simulink model "task4_neo"  (Simulink 8.3)
settings: Solver=ode45  StartTime=0.0  StopTime=250  RelTol=1e-3
PreLoadFcn:
  | % Nelson Campos
  | 
  | clear all
  | close all
  | 
  | s = tf('s');
  | 
  | H = tf(1, [100 20 1], 'InputDelay', 1);
  | 
  | 
  | Kc = 15;
  | Ti = 6.75;
  | Td = 1.69;
  | 
  | PID = [Kc Ti Td];
  | Gc = PID(1)*(1+1/(PID(2)*s)+PID(3)*s);
  | 
  | i, F = feedback(Gc*H,1);
  | [y,t] = step(F);
  | 
  | 
  | Features = calculateFeatures(F,y,t);
InitFcn:
  | Ku = 25;
  | Tu = 13.5;
  | Kpmin = 0.55*Ku;
  | Kpmax = 0.65*Ku;
  | Kdmin = 0.12*Ku*Tu;
  | Kdmax = 0.16*Ku*Tu;
  | Kimin = 1.9*Ku/Tu;
  | Kimax = 2.1*Ku/Tu;
  | 
  | fuzzy_final3 = readfis('fuzzy_sugeno_pid');
values from neighbouring files (symbols this model uses):
  F = feedback(Gc*H,1)    [task4_m.m]
libraries: fuzblock x1
settings Model: Creator=erobotica  LastModifiedBy=erobotica
settings DataIOCC: SignalLoggingSaveFormat=Dataset
settings DebuggingCC: UnderspecifiedInitializationDetection=Simplified  StateNameClashWarn=none
settings GRTTargetCC: CombineOutputUpdateFcns=on  GRTInterface=off

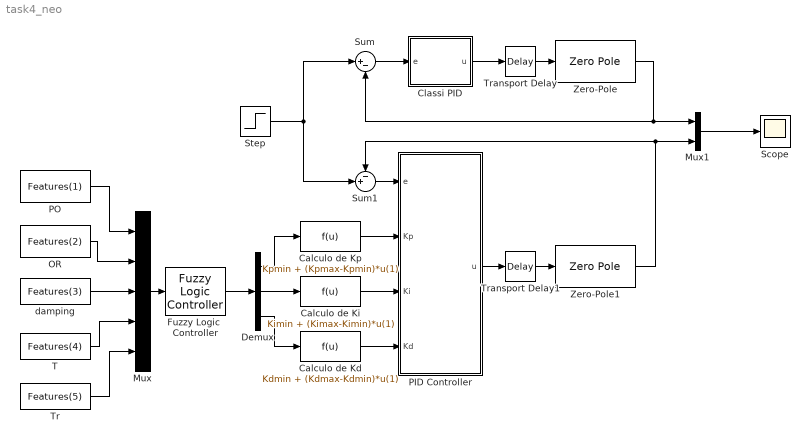
== system task4_neo ==
  Calculo de Kd : Fcn  Expr=Kdmin + (Kdmax-Kdmin)*u(1)
  Calculo de Ki : Fcn  Expr=Kimin + (Kimax-Kimin)*u(1)
  Calculo de Kp : Fcn  Expr=Kpmin + (Kpmax-Kpmin)*u(1)
  Classi PID : Subsystem
  Demux : Demux  Outputs=3
  Fuzzy Logic  Controller : fuzblock/Fuzzy Logic  Controller  fis=fuzzy_final3
  Mux : Mux  Inputs=5
  Mux1 : Mux  Inputs=2
  OR : Constant  Value=Features(2)
  PID Controller : Subsystem
  PO : Constant  Value=Features(1)
  Scope : Scope
      settings: TimeRange=250  YMin=-2.214156079854803  YMax=3.393829401088933
  Step : Step  Time=0  SampleTime=0.1
  Sum : Sum  Inputs=|+-
  Sum1 : Sum  Inputs=-+|
  T : Constant  Value=Features(4)
  Tr : Constant  Value=Features(5)
  Transport Delay : TransportDelay  DelayTime=0.5
  Transport Delay1 : TransportDelay  DelayTime=0.5
  Zero-Pole : ZeroPole  Zeros=[]  Poles=[-0.1 -0.1]  Gain=0.01
  Zero-Pole1 : ZeroPole  Zeros=[]  Poles=[-0.1 -0.1]  Gain=0.01
  damping : Constant  Value=Features(3)
  wires:
  Transport Delay/1 -> Zero-Pole/1
  Classi PID/1(u) -> Transport Delay/1
  Sum/1 -> Classi PID/1(e)
  Mux1/1 -> Scope/1
  Step/1 -> Sum/1, Sum1/2
  PO/1 -> Mux/1
  Tr/1 -> Mux/5
  Zero-Pole/1 -> Mux1/1, Sum/2
  Transport Delay1/1 -> Zero-Pole1/1
  PID Controller/1(u) -> Transport Delay1/1
  Zero-Pole1/1 -> Sum1/1, Mux1/2
  Mux/1 -> Fuzzy Logic  Controller/1
  damping/1 -> Mux/3
  OR/1 -> Mux/2
  T/1 -> Mux/4
  Fuzzy Logic  Controller/1 -> Demux/1
  Demux/1 -> Calculo de Kp/1
  Demux/3 -> Calculo de Kd/1
  Demux/2 -> Calculo de Ki/1
  Calculo de Kp/1 -> PID Controller/2(Kp)
  Calculo de Ki/1 -> PID Controller/3(Ki)
  Calculo de Kd/1 -> PID Controller/4(Kd)
  Sum1/1 -> PID Controller/1(e)

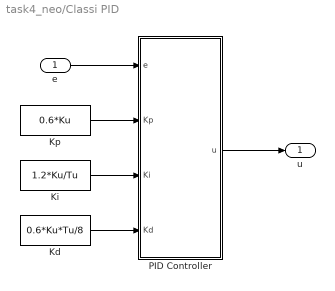
== system task4_neo/Classi PID ==
  e : Inport
  Kd : Constant  Value=0.6*Ku*Tu/8
  Ki : Constant  Value=1.2*Ku/Tu
  Kp : Constant  Value=0.6*Ku
  PID Controller : Subsystem
  u : Outport
  wires:
  Kd/1 -> PID Controller/4(Kd)
  PID Controller/1(u) -> u/1
  e/1 -> PID Controller/1(e)
  Kp/1 -> PID Controller/2(Kp)
  Ki/1 -> PID Controller/3(Ki)

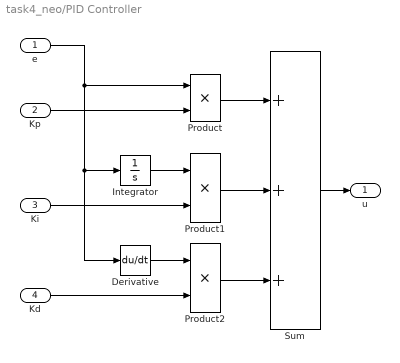
== system task4_neo/PID Controller ==
  e : Inport
  Kp : Inport  Port=2
  Ki : Inport  Port=3
  Kd : Inport  Port=4
  Derivative : Derivative
  Integrator : Integrator
  Product : Product
  Product1 : Product
  Product2 : Product
  Sum : Sum  Inputs=3
  u : Outport
  wires:
  Sum/1 -> u/1
  Product/1 -> Sum/1
  Kp/1 -> Product/2
  e/1 -> Derivative/1, Integrator/1, Product/1
  Ki/1 -> Product1/2
  Integrator/1 -> Product1/1
  Product1/1 -> Sum/2
  Product2/1 -> Sum/3
  Kd/1 -> Product2/2
  Derivative/1 -> Product2/1

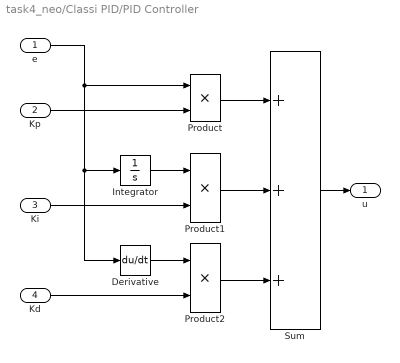
== system task4_neo/Classi PID/PID Controller ==
  e : Inport
  Kp : Inport  Port=2
  Ki : Inport  Port=3
  Kd : Inport  Port=4
  Derivative : Derivative
  Integrator : Integrator
  Product : Product
  Product1 : Product
  Product2 : Product
  Sum : Sum  Inputs=3
  u : Outport
  wires:
  Sum/1 -> u/1
  Product/1 -> Sum/1
  Kp/1 -> Product/2
  e/1 -> Derivative/1, Integrator/1, Product/1
  Ki/1 -> Product1/2
  Integrator/1 -> Product1/1
  Product1/1 -> Sum/2
  Product2/1 -> Sum/3
  Kd/1 -> Product2/2
  Derivative/1 -> Product2/1
